simulink model "practice1"  (R2023a)
settings: Solver=VariableStepAuto  StartTime=0.0  StopTime=10  RelTol=1e-3
settings Model: PauseTimes=10  Creator=fxin  LastModifiedBy=fxin

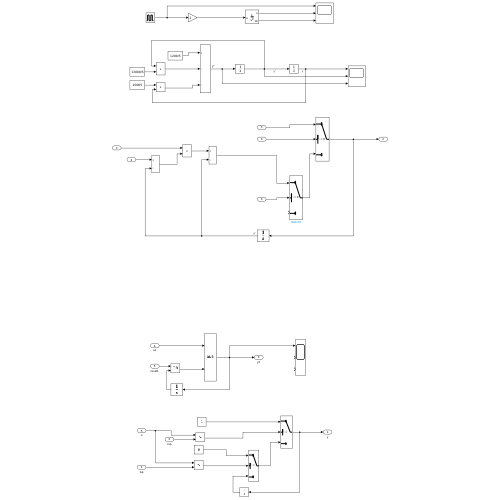
[thumbnail: Simulink's stored preview of the top-level diagram]
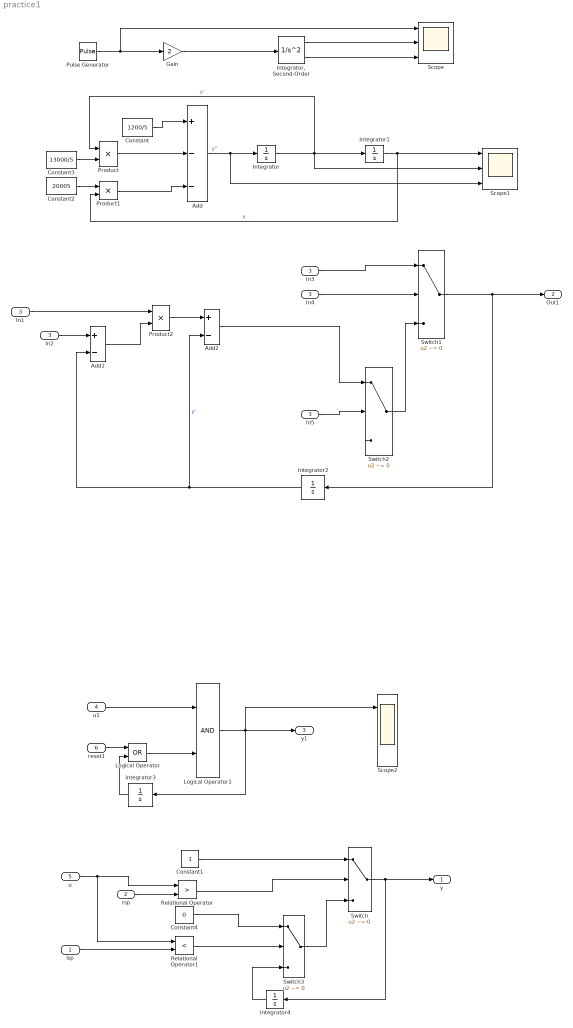
== system practice1 ==
  note: y''
  lsp : Inport
  rsp : Inport  Port=2
  In1 : Inport  Port=3
  u1 : Inport  Port=4
  u : Inport  Port=5
  reset1 : Inport  Port=6
  Add : Sum  Inputs=+--
  Add1 : Sum  Inputs=+-
  Add2 : Sum  Inputs=+-
  Constant : Constant  Value=1200/5
  Constant1 : Constant
  Constant2 : Constant  Value=20005
  Constant3 : Constant  Value=13000/5
  Constant4 : Constant  Value=0
  Gain : Gain  Gain=2
  In{2..5} (4 alike) : InportShadow  Port=3
  Integrator{,1..4} (5 alike) : Integrator
  "Integrator, Second-Order" : SecondOrderIntegrator
  Logical Operator : Logic  Operator=OR  AllPortsSameDT=off  OutDataTypeStr=boolean
  Logical Operator1 : Logic  AllPortsSameDT=off  OutDataTypeStr=boolean
  Product : Product
  Product1 : Product
  Product2 : Product
  Pulse Generator : DiscretePulseGenerator  PulseType=Time based  Period=10  PulseWidth=5
  Relational Operator : RelationalOperator  Operator=>  OutDataTypeStr=boolean  RndMeth=Simplest  InputSameDT=off
  Relational Operator1 : RelationalOperator  Operator=<  OutDataTypeStr=boolean  RndMeth=Simplest  InputSameDT=off
  Scope : Scope  NumInputPorts=3
  Scope1 : Scope  NumInputPorts=3
  Scope2 : Scope  NumInputPorts=3
  Switch{,1..3} (4 alike) : Switch  Criteria=u2 ~= 0  SaturateOnIntegerOverflow=off  InputSameDT=off
  y : Outport
  Out1 : Outport  Port=2
  y1 : Outport  Port=3
  wires:
  Pulse Generator/1 -> Scope/1, Gain/1
  Gain/1 -> "Integrator, Second-Order"/1
  "Integrator, Second-Order"/1 -> Scope/2
  "Integrator, Second-Order"/2 -> Scope/3
  Add/1 -> Integrator/1, Scope1/3
  Integrator/1 -> Product/1, Scope1/2, Integrator1/1  "y'"
  Integrator1/1 -> Scope1/1, Product1/2  "y"
  Constant/1 -> Add/1
  Product/1 -> Add/2
  Constant2/1 -> Product1/1
  Product1/1 -> Add/3
  Constant3/1 -> Product/2
  In2/1 -> Add1/1
  In1/1 -> Product2/1
  Add1/1 -> Product2/2
  Product2/1 -> Add2/1
  Add2/1 -> Switch2/1
  In5/1 -> Switch2/2
  In3/1 -> Switch1/1
  In4/1 -> Switch1/2
  Switch2/1 -> Switch1/3
  Switch1/1 -> Integrator2/1, Out1/1
  Integrator2/1 -> Add2/2, Add1/2  "y'"
  reset1/1 -> Logical Operator/1
  u1/1 -> Logical Operator1/1
  Logical Operator/1 -> Logical Operator1/2
  Logical Operator1/1 -> Scope2/1, Integrator3/1, y1/1
  Integrator3/1 -> Logical Operator/2
  Constant1/1 -> Switch/1
  u/1 -> Relational Operator1/1, Relational Operator/1
  rsp/1 -> Relational Operator/2
  Relational Operator/1 -> Switch/2
  Constant4/1 -> Switch3/1
  Relational Operator1/1 -> Switch3/2
  Switch3/1 -> Switch/3
  lsp/1 -> Relational Operator1/2
  Integrator4/1 -> Switch3/3
  Switch/1 -> Integrator4/1, y/1
